simulink model "Motor2_Avellaneda"  (R2023b)
settings: Solver=VariableStepAuto  StartTime=0.0  StopTime=3  RelTol=1e-3
settings Model: Creator=Usuario  LastModifiedBy=Usuario

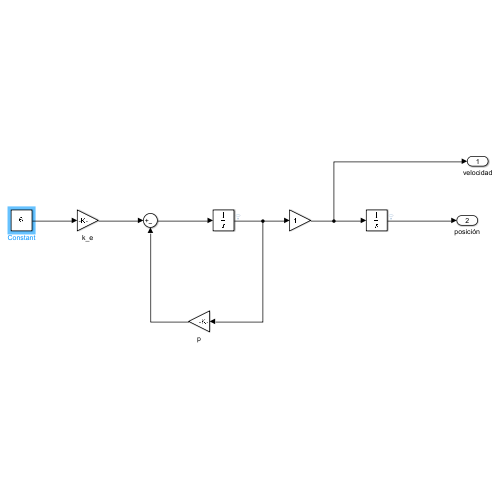
[thumbnail: Simulink's stored preview of the top-level diagram]
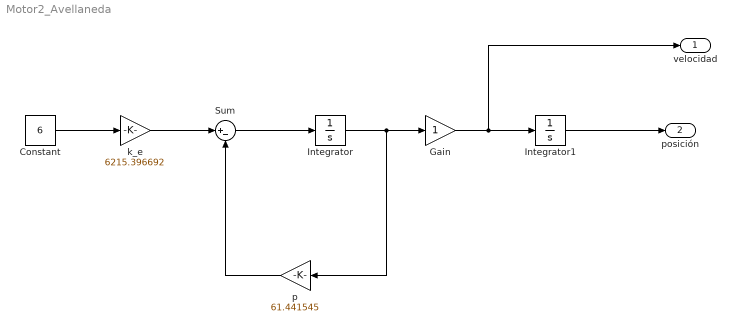
== system Motor2_Avellaneda ==
  Constant : Constant  Value=6
  Gain : Gain
  Integrator : Integrator
  Integrator1 : Integrator
  Sum : Sum  Inputs=|+-
  k_e : Gain  Gain=6215.396692
  p : Gain  Gain=61.441545
  velocidad : Outport
  posición : Outport  Port=2
  wires:
  Constant/1 -> k_e/1
  k_e/1 -> Sum/1
  Sum/1 -> Integrator/1
  Integrator/1 -> p/1, Gain/1
  Gain/1 -> velocidad/1, Integrator1/1
  p/1 -> Sum/2
  Integrator1/1 -> posición/1
